simulink model "rtwdemo_roll_Step02a"  (R2022b)
settings: Solver=FixedStepDiscrete  StartTime=0.0  StopTime=30  FixedStep=0.025  RelTol=1e-3
model workspace (MATLAB code in the model file + MAT data in the model file):
  | cmdLim = Simulink.Parameter;
  | cmdLim.Value = 15;
  | cmdLim.Description = 'Limit for controlling the maximum surface command angle.';
  | cmdLim.Min = 0;
  | cmdLim.Max = 90;
  | cmdLim.DocUnits = 'deg';
  | 
  | dispGain = Simulink.Parameter;
  | dispGain.Value = 0.75;
  | dispGain.Description = 'Gain applied to the displacement error.';
  | dispGain.Min = 0;
  | dispGain.Max = [];
  | dispGain.DocUnits = 'deg/sec/deg';
  | 
  | dispLim = Simulink.Parameter;
  | dispLim.Value = 30;
  | dispLim.Description = 'Limit for controlling the maximum commanded angle.';
  | dispLim.Min = 0;
  | dispLim.Max = 180;
  | dispLim.DocUnits = 'deg';
  | 
  | intGain = Simulink.Parameter;
  | intGain.Value = 0.5;
  | intGain.Description = 'Gain applied to the integral error.';
  | intGain.Min = 0;
  | intGain.Max = [];
  | intGain.DocUnits = 'deg/sec/deg/sec';
  | 
  | intLim = Simulink.Parameter;
  | intLim.Value = 5;
  | intLim.Description = 'Limit for controlling the maximum commanded angle.';
  | intLim.Min = 0;
  | intLim.Max = 90;
  | intLim.DocUnits = 'deg';
  | 
  | rateGain = Simulink.Parameter;
  | rateGain.Value = 2;
  | rateGain.Description = 'Gain applied to the rate error.';
  | rateGain.Min = 0;
  | rateGain.Max = [];
  | rateGain.DocUnits = 'deg/deg/sec';
  | 
  | rateLim = Simulink.Parameter;
  | rateLim.Value = 6;
  | rateLim.Description = 'Limit for controlling the maximum commanded angle.';
  | rateLim.Min = 0;
  | rateLim.Max = 180;
  | rateLim.DocUnits = 'deg/sec';
  | 
  | hdgGain = Simulink.Parameter;
  | hdgGain.Value = 0.015;
undefined symbols (not defined in the file): DiscIntNeverNeededParam
libraries: simulink_need_slupdate x1
Description:
  | This model represents a basic roll axis autopilot with two operating
  | modes; roll attitude hold and heading hold. The mode logic for these
  | modes is external to this model.  The model architecture represents the
  | heading hold mode and basic roll attitude function as referenced models.
  | 
  | The roll attitude control function is a PID controller that uses roll
  | attitude and roll rate feedback to produce an aileron command.  The
  | input to the controller will be either a basic roll angle reference or a
  | roll command to track the desired heading.
settings Model: RequirementInfo={} %GIDa_fe9045fd_0412_4b6e_8206_617cc20e6fde  FPTRunName=Active  ModifiedByFormat=The MathWorks, Inc.  Creator=The MathWorks, Inc.  LastModifiedBy=The MathWorks, Inc.
settings SolverCC: AlgebraicLoopSolver=TrustRegion
settings DataIOCC: ExternalInput=xin  SaveFormat=StructureWithTime  SaveOutput=off  SignalLogging=off  DSMLogging=off  SaveTime=off  ReturnWorkspaceOutputs=off
settings OptimizationCC: UseDivisionForNetSlopeComputation=on  UseFloatMulNetSlope=on  EnhancedBackFolding=on  BooleansAsBitfields=on  PassReuseOutputArgsAs=Individual arguments  ExpressionDepthLimit=2147483647  NoFixptDivByZeroProtection=on  EfficientFloat2IntCast=on  MaxStackSize=inf  OptimizeBlockOrder=speed  DifferentSizesBufferReuse=on  EfficientTunableParamExpr=on
settings DebuggingCC: SignalRangeChecking=error  ReadBeforeWriteMsg=EnableAllAsError  WriteAfterWriteMsg=EnableAllAsError  WriteAfterReadMsg=EnableAllAsError  AlgebraicLoopMsg=error  ArtificialAlgebraicLoopMsg=error  SaveWithDisabledLinksMsg=error  SaveWithParameterizedLinksMsg=error  CheckExecutionContextPreStartOutputMsg=on  BlockPriorityViolationMsg=error  MaxConsecutiveZCsMsg=warning  SolverPrmCheckMsg=error  InheritedTsInSrcMsg=error  SingleTaskRateTransMsg=error  TasksWithSamePriorityMsg=error  SigSpecEnsureSampleTimeMsg=error  IntegerOverflowMsg=error  ParameterUnderflowMsg=error  ParameterPrecisionLossMsg=none  ParameterTunabilityLossMsg=error  UnderSpecifiedDataTypeMsg=error  UnnecessaryDatatypeConvMsg=warning  VectorMatrixConversionMsg=error  SignalLabelMismatchMsg=error  UnconnectedInputMsg=error  UnconnectedOutputMsg=error  UnconnectedLineMsg=error  SFcnCompatibilityMsg=error  UniqueDataStoreMsg=error  BusObjectLabelMismatch=error  RootOutportRequireBusObject=error  AssertControl=DisableAll  AllowSymbolicDim=off  ModelReferenceIOMsg=error  ModelReferenceIOMismatchMessage=error  UnknownTsInhSupMsg=error  ModelReferenceDataLoggingMessage=error  ModelReferenceSymbolNameMessage=none  ModelReferenceExtraNoncontSigs=none  StateNameClashWarn=warning  StrictBusMsg=ErrorOnBusTreatedAsVector  NonBusSignalsTreatedAsBus=error  SFInvalidInputDataAccessInChartInitDiag=error  SFTransitionOutsideNaturalParentDiag=error  SFUnreachableExecutionPathDiag=error  SFUndirectedBroadcastEventsDiag=error  SFExecutionAtInitializationDiag=none  SFMachineParentedDataDiag=warning  IntegerSaturationMsg=error  ArithmeticOperatorsInVariantConditions=warning
settings HardwareCC: ProdLongLongMode=on  TargetHWDeviceType=32-bit Generic
settings ModelReferenceCC: EnableRefExpFcnMdlSchedulingChecks=on  ModelReferenceNumInstancesAllowed=Single  PropagateSignalLabelsOutOfModel=off
settings SFSimCC: SimUseLocalCustomCode=off  MATLABDynamicMemAlloc=off
settings RTWCC: Description=Embedded Coder  SystemTargetFile=ert.tlc  GenCodeOnly=on  TemplateMakefile=ert_default_tmf  GenerateReport=on  RTWVerbose=off  RTWUseLocalCustomCode=off  CustomSource=roll_input_data.c  BuildConfiguration=Faster Runs  IncludeHyperlinkInReport=on  LaunchReport=on  GenerateTraceInfo=on  GenerateTraceReport=on  GenerateTraceReportSl=on  GenerateTraceReportSf=on  GenerateTraceReportEml=on  GenerateCodeMetricsReport=on  DLArmComputeVersion=19.05
settings CodeAppCC: ForceParamTrailComments=on  IgnoreCustomStorageClasses=off  OperatorAnnotations=on  SimulinkDataObjDesc=on  SFDataObjDesc=on  CustomSymbolStrGlobalVar=$N$M  CustomSymbolStrType=$N$M  CustomSymbolStrFcn=$N$M$F  CustomSymbolStrMacro=$N$M  InsertBlockDesc=on  ReqsInCode=on
settings ERTTargetCC: GenerateSampleERTMain=on  ERTCustomFileTemplate=example_file_process.tlc
settings ConfigComp: CovScope=ReferencedModels  CovSaveName=covdata_rollAP  CovMetricSettings=dcmtrwe  CovHTMLOptions=-sRT=1 -aTS=1 -bRG=1 -bTC=1 -hTR=1 -nFC=0 -scm=1 -bcm=1 -xEv=0  CovSaveCumulativeToWorkspaceVar=on  CovSaveSingleToWorkspaceVar=on  CovCumulativeVarName=covCumulativeData_rollAP  CovReportOnPause=off  CovExternalEMLEnable=off  CovSFcnEnable=off  DVModelCoverageObjectives=MCDC  DVMaxTestCaseSteps=500  DVTestSuiteOptimization=CombinedObjectives (Nonlinear Extended)  DVDetectActiveLogic=on  DVSaveHarnessModel=on  DVModelReferenceHarness=on  DVSaveReport=on  DVRebuildModelRepresentation=Always

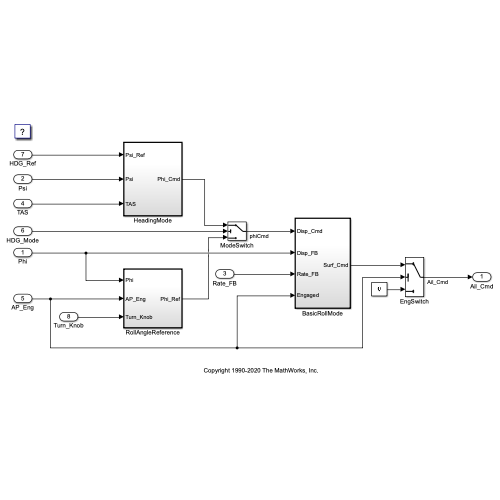
[thumbnail: Simulink's stored preview of the top-level diagram]
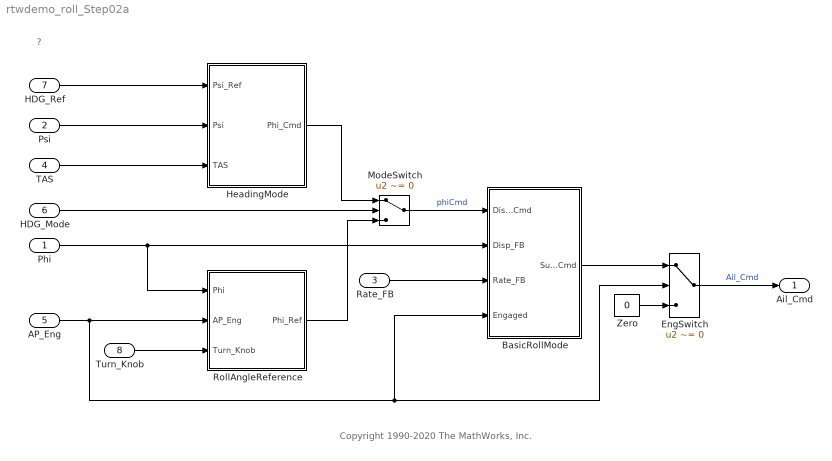
== system rtwdemo_roll_Step02a ==
  note: Copyright 1990-2020 The MathWorks, Inc.
  note: ?
  Phi : Inport  RequirementInfo={} %GIDa_040c2d73_6311_42f9_964f_56f1fff3d8d8  OutMin=-180  OutMax=180  OutDataTypeStr=single  PortDimensions=1  SampleTime=1/40  Interpolate=off
  Psi : Inport  RequirementInfo={} %GIDa_aa699f91_96f0_401b_acdb_f9b4b0743533  Port=2  OutMin=-180  OutMax=180  OutDataTypeStr=single  PortDimensions=1  SampleTime=1/40  Interpolate=off
  Rate_FB : Inport  RequirementInfo={} %GIDa_91b6e343_cedd_4c09_9e82_9cc09e4312a7  Port=3  OutMin=-60  OutMax=60  OutDataTypeStr=single  PortDimensions=1  SampleTime=1/40  Interpolate=off
  TAS : Inport  RequirementInfo={} %GIDa_9daa2c3d_09c1_4ac6_a206_1425f5f778cd  Port=4  OutMin=0  OutMax=1000  OutDataTypeStr=single  PortDimensions=1  SampleTime=1/40  Interpolate=off
  AP_Eng : Inport  RequirementInfo={} %GIDa_dbf8c750_871c_42fc_8ea1_57838e97fa97  Port=5  OutMin=0  OutMax=1  OutDataTypeStr=boolean  PortDimensions=1  SampleTime=1/40  Interpolate=off
  HDG_Mode : Inport  RequirementInfo={} %GIDa_3d1fd2be_b046_42ef_8f3c_1955bceadbb7  Port=6  OutMin=0  OutMax=1  OutDataTypeStr=boolean  PortDimensions=1  SampleTime=1/40  Interpolate=off
  HDG_Ref : Inport  RequirementInfo={} %GIDa_96162cda_cb1a_490e_8dac_f861526aad50  Port=7  OutMin=-180  OutMax=180  OutDataTypeStr=single  PortDimensions=1  SampleTime=1/40  Interpolate=off
  Turn_Knob : Inport  RequirementInfo={} %GIDa_fa976ccd_1ea9_4823_b673_fef2768ad601  Port=8  OutMin=-45  OutMax=45  OutDataTypeStr=single  PortDimensions=1  SampleTime=1/40  Interpolate=off
  BasicRollMode : Subsystem  TreatAsAtomicUnit=on
      settings: RTWSystemCode=Inline
  EngSwitch : Switch  RequirementInfo={} %GIDa_1f89e2a1_f10b_411b_80f1_4c7070559f04  Criteria=u2 ~= 0  OutDataTypeStr=single  SaturateOnIntegerOverflow=off  InputSameDT=off
  HeadingMode : Subsystem  TreatAsAtomicUnit=on
      settings: RTWSystemCode=Inline
  ModeSwitch : Switch  RequirementInfo={} %GIDa_89518de0_411a_4ee8_869d_c7ed5e5087e3  Criteria=u2 ~= 0  OutDataTypeStr=single  SaturateOnIntegerOverflow=off  InputSameDT=off
  RollAngleReference : Subsystem  RequirementInfo={} %GIDa_bf621fce_78e1_4f75_9fdb_aa952a465c6d  TreatAsAtomicUnit=on
      settings: RTWSystemCode=Inline
  Zero : Constant  RequirementInfo={} %GIDa_8c99e557_6257_4659_beae_770a67a6ac3a  Value=0  OutDataTypeStr=single
  Ail_Cmd : Outport  RequirementInfo={} %GIDa_02b61f6d_71d4_4b0d_89ac_bfbca808eb5f  OutMin=-15  OutMax=15  OutDataTypeStr=single  PortDimensions=1  SampleTime=1/40  VectorParamsAs1DForOutWhenUnconnected=off
  wires:
  HDG_Ref/1 -> HeadingMode/1(Psi_Ref)
  Phi/1 -> RollAngleReference/1(Phi), BasicRollMode/2(Disp_FB)
  Rate_FB/1 -> BasicRollMode/3(Rate_FB)
  Psi/1 -> HeadingMode/2(Psi)
  TAS/1 -> HeadingMode/3(TAS)
  ModeSwitch/1 -> BasicRollMode/1(Disp_Cmd)  "phiCmd"
  HDG_Mode/1 -> ModeSwitch/2
  HeadingMode/1(Phi_Cmd) -> ModeSwitch/1
  AP_Eng/1 -> BasicRollMode/4(Engaged), EngSwitch/2, RollAngleReference/2(AP_Eng)
  BasicRollMode/1(Surf_Cmd) -> EngSwitch/1
  EngSwitch/1 -> Ail_Cmd/1  "Ail_Cmd"
  Zero/1 -> EngSwitch/3
  RollAngleReference/1(Phi_Ref) -> ModeSwitch/3
  Turn_Knob/1 -> RollAngleReference/3(Turn_Knob)

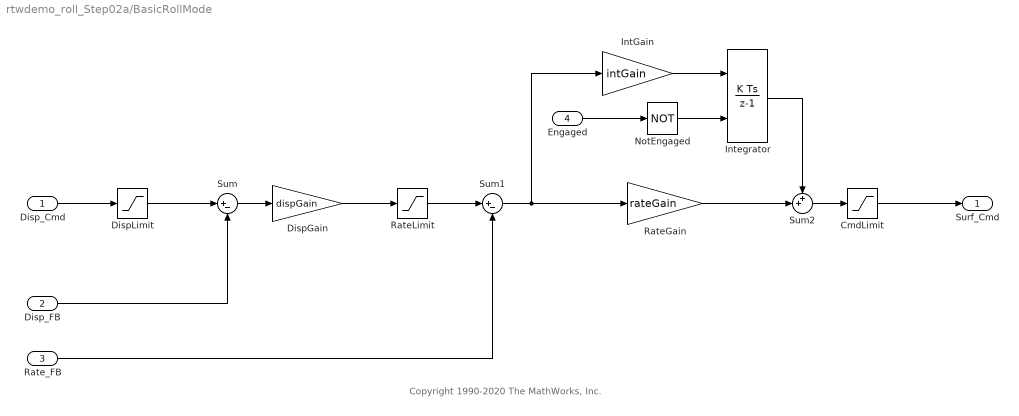
== system rtwdemo_roll_Step02a/BasicRollMode ==
  note: Copyright 1990-2020 The MathWorks, Inc.
  Disp_Cmd : Inport  RequirementInfo={} %GIDa_ff8f2950_36d2_4703_9842_3782e1cf4043  OutMin=-180  OutMax=180  OutDataTypeStr=single  PortDimensions=1  SampleTime=1/40
  Disp_FB : Inport  RequirementInfo={} %GIDa_88ab7783_4881_4494_98c7_fae9a40f845a  Port=2  OutMin=-180  OutMax=180  OutDataTypeStr=single  PortDimensions=1  SampleTime=1/40
  Rate_FB : Inport  RequirementInfo={} %GIDa_4b3300d7_83b5_4816_b86c_8919c709dd87  Port=3  OutMin=-60  OutMax=60  OutDataTypeStr=single  PortDimensions=1  SampleTime=1/40
  Engaged : Inport  RequirementInfo={} %GIDa_68912e61_3a66_45a7_b507_2a909d737c47  Port=4  OutMin=0  OutMax=1  OutDataTypeStr=boolean  PortDimensions=1  SampleTime=1/40
  CmdLimit : Saturate  RequirementInfo={} %GIDa_03acfcd2_0166_4b8d_8424_6cefd1433742  UpperLimit=cmdLim  LowerLimit=-cmdLim
      settings: AttributesFormatString=%<LowerLimit> to %<UpperLimit>\n(deg)
  DispGain : Gain  RequirementInfo={} %GIDa_dff0c99b_8bb2_4fb9_8fd5_e82c46b12065  Gain=dispGain  OutDataTypeStr=Inherit: Same as input  ParamDataTypeStr=Inherit: Same as input
  DispLimit : Saturate  RequirementInfo={} %GIDa_b12ad7d0_7f46_4ac9_8f07_3dc9a608e0b9  UpperLimit=dispLim  LowerLimit=-dispLim  OutMin=-dispLim  OutMax=dispLim
      settings: AttributesFormatString=%<LowerLimit> to %<UpperLimit>\n(deg)
  IntGain : Gain  RequirementInfo={} %GIDa_b5140734_8c8b_40a9_9825_d7d1205e8869  Gain=intGain  OutDataTypeStr=Inherit: Same as input  ParamDataTypeStr=Inherit: Same as input
  Integrator : DiscreteIntegrator  RequirementInfo={} %GIDa_4ed31261_78e4_4834_bce8_809b2d91a32f  ExternalReset=level  SampleTime=1/40  OutMin=-intLim  OutMax=intLim  OutDataTypeStr=single  LimitOutput=on  UpperSaturationLimit=intLim  LowerSaturationLimit=-intLim  IgnoreLimit=on  ICPrevOutput=DiscIntNeverNeededParam  ICPrevScaledInput=DiscIntNeverNeededParam
      settings: AttributesFormatString=%<LowerSaturationLimit> to %<UpperSaturationLimit> (deg)
  NotEngaged : Logic  RequirementInfo={} %GIDa_708249e7_acd0_4b17_bb48_cb1f255fa1ae  Operator=NOT  IconShape=distinctive  AllPortsSameDT=off  OutDataTypeStr=boolean
  RateGain : Gain  RequirementInfo={} %GIDa_1d522638_1084_40aa_a9e2_d20f3b201758  Gain=rateGain  OutDataTypeStr=Inherit: Same as input  ParamDataTypeStr=Inherit: Same as input
  RateLimit : Saturate  RequirementInfo={} %GIDa_3a07b6bd_f8e9_4edb_b789_30fb5da492d2  UpperLimit=rateLim  LowerLimit=-rateLim  OutMin=-rateLim  OutMax=rateLim
      settings: AttributesFormatString=%<LowerLimit> to %<UpperLimit>\n(deg/sec)
  Sum : Sum  RequirementInfo={} %GIDa_ed2635df_4414_4276_958f_e2737d50d7e7  Inputs=|+-  AccumDataTypeStr=single  OutDataTypeStr=single
  Sum1 : Sum  RequirementInfo={} %GIDa_c2525d12_4b8c_459a_a1b7_e9245b378d44  Inputs=|+-  AccumDataTypeStr=single  OutDataTypeStr=single
  Sum2 : Sum  RequirementInfo={} %GIDa_6cc23380_db4c_4d56_bea9_1d957a833aee  Inputs=++|  AccumDataTypeStr=single  OutDataTypeStr=single
  Surf_Cmd : Outport  RequirementInfo={} %GIDa_f913a5d7_0f1c_420b_9466_7f1cf663aa04  OutMin=-cmdLim  OutMax=cmdLim  OutDataTypeStr=single  PortDimensions=1  SampleTime=1/40  VectorParamsAs1DForOutWhenUnconnected=off
  wires:
  Disp_Cmd/1 -> DispLimit/1
  Disp_FB/1 -> Sum/2
  Rate_FB/1 -> Sum1/2
  Sum1/1 -> RateGain/1, IntGain/1
  DispGain/1 -> RateLimit/1
  Sum/1 -> DispGain/1
  DispLimit/1 -> Sum/1
  RateLimit/1 -> Sum1/1
  CmdLimit/1 -> Surf_Cmd/1
  RateGain/1 -> Sum2/2
  Sum2/1 -> CmdLimit/1
  Engaged/1 -> NotEngaged/1
  NotEngaged/1 -> Integrator/2
  Integrator/1 -> Sum2/1
  IntGain/1 -> Integrator/1

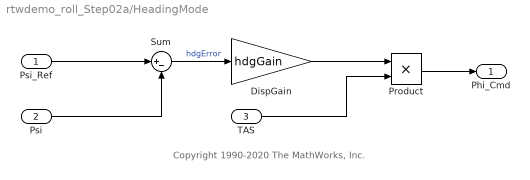
== system rtwdemo_roll_Step02a/HeadingMode ==
  note: Copyright 1990-2020 The MathWorks, Inc.
  Psi_Ref : Inport  RequirementInfo={} %GIDa_63217851_dfde_4515_9b44_03620ba74ebd  OutMin=-180  OutMax=180  OutDataTypeStr=single  PortDimensions=1  SampleTime=1/40  Interpolate=off
  Psi : Inport  RequirementInfo={} %GIDa_fd436e7a_0b55_4fc9_b9d1_7e931e78faf3  Port=2  OutMin=-180  OutMax=180  OutDataTypeStr=single  PortDimensions=1  SampleTime=1/40  Interpolate=off
  TAS : Inport  RequirementInfo={} %GIDa_5afcdc4c_2f58_40a9_83dd_f8ee574f1321  Port=3  OutMin=0  OutMax=1000  OutDataTypeStr=single  PortDimensions=1  SampleTime=1/40  Interpolate=off
  DispGain : Gain  RequirementInfo={} %GIDa_efcf24d9_d92c_4e12_9177_4c044d8f8aec  Gain=hdgGain  OutDataTypeStr=Inherit: Same as input  ParamDataTypeStr=Inherit: Same as input
  Product : Product  RequirementInfo={} %GIDa_7dbe21d3_99ef_4184_ab1e_23ac1efc2950  RndMeth=Zero  OutDataTypeStr=Inherit: Same as first input
  Sum : Sum  RequirementInfo={} %GIDa_3ad2d5f4_d194_4ab5_91b1_326f1f050e43  Inputs=|+-  OutDataTypeStr=Inherit: Same as first input
  Phi_Cmd : Outport  RequirementInfo={} %GIDa_6cfb4d70_f1fd_4187_9f6e_37a982bfddd8  OutDataTypeStr=single  PortDimensions=1  SampleTime=1/40  VectorParamsAs1DForOutWhenUnconnected=off
  wires:
  Product/1 -> Phi_Cmd/1
  DispGain/1 -> Product/1
  Sum/1 -> DispGain/1  "hdgError"
  Psi/1 -> Sum/2
  Psi_Ref/1 -> Sum/1
  TAS/1 -> Product/2

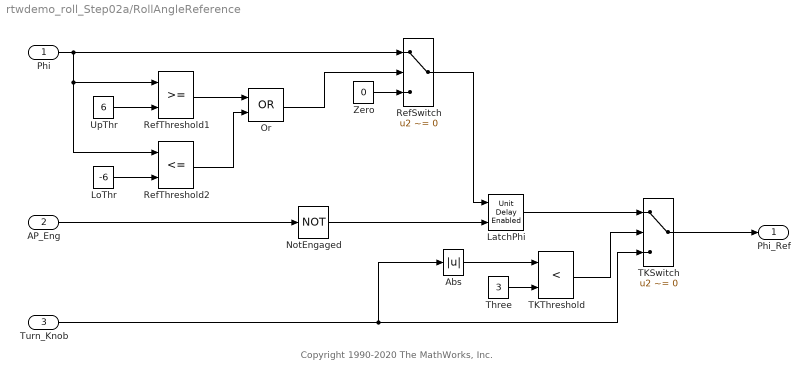
== system rtwdemo_roll_Step02a/RollAngleReference ==
  note: Copyright 1990-2020 The MathWorks, Inc.
  Phi : Inport  RequirementInfo={} %GIDa_9b709a66_f791_47f7_86bd_e175ebb7b1b4  OutDataTypeStr=single
  AP_Eng : Inport  RequirementInfo={} %GIDa_9de52ebb_3f37_4f5e_876e_6853370267c1  Port=2  OutDataTypeStr=boolean
  Turn_Knob : Inport  RequirementInfo={} %GIDa_fcc46fb4_e425_442f_ac5c_e3f314b4cbdd  Port=3  OutDataTypeStr=single
  Abs : Abs  RequirementInfo={} %GIDa_daf2388c_0592_4fd8_9932_fc6ad2b28c75  SaturateOnIntegerOverflow=off
  LatchPhi : simulink_need_slupdate/Unit Delay Enabled  RequirementInfo={} %GIDa_8c2a6474_62f7_4673_9b80_815aaee792d7  vinit=0.0  tsamp=1/40
  LoThr : Constant  RequirementInfo={} %GIDa_3d290e71_7846_48ec_bba2_120ec195a4d2  Value=-6  OutDataTypeStr=single
  NotEngaged : Logic  RequirementInfo={} %GIDa_e52c6893_d81b_4f15_89c3_12b6a83c27b2  Operator=NOT  IconShape=distinctive  AllPortsSameDT=off  OutDataTypeStr=boolean
  Or : Logic  RequirementInfo={} %GIDa_5a2f4265_d6d2_48b0_88b1_9f813e67f638  Operator=OR  OutDataTypeStr=boolean
  RefSwitch : Switch  RequirementInfo={} %GIDa_a4746381_6ebe_4e3d_83b9_b49d14a3af5e  Criteria=u2 ~= 0  OutDataTypeStr=single  SaturateOnIntegerOverflow=off  InputSameDT=off
  RefThreshold1 : RelationalOperator  RequirementInfo={} %GIDa_be19764a_4253_499a_816c_5a218f85ba52  OutDataTypeStr=boolean
  RefThreshold2 : RelationalOperator  RequirementInfo={} %GIDa_66db49a9_aa40_43ab_9d6f_efe68ac443ed  Operator=<=  OutDataTypeStr=boolean
  TKSwitch : Switch  RequirementInfo={} %GIDa_804165d0_89eb_4919_a8d1_f2310004f7d9  Criteria=u2 ~= 0  OutDataTypeStr=single  SaturateOnIntegerOverflow=off  InputSameDT=off
  TKThreshold : RelationalOperator  RequirementInfo={} %GIDa_9859b478_272f_4974_a36c_6c4f8c030643  Operator=<  OutDataTypeStr=boolean
  Three : Constant  RequirementInfo={} %GIDa_6228e2c4_8022_4eaf_90d6_7c47f19fb0a2  Value=3  OutDataTypeStr=single
  UpThr : Constant  RequirementInfo={} %GIDa_0870d8d6_d29f_4cb4_9c0c_9079ccdb7173  Value=6  OutDataTypeStr=single
  Zero : Constant  RequirementInfo={} %GIDa_e4775650_e5c7_4c74_aef4_71c144af3cbc  Value=0  OutDataTypeStr=single
  Phi_Ref : Outport  RequirementInfo={} %GIDa_130f2b33_9208_4d69_9109_0436e6034ad0  OutMin=-180  OutMax=180  OutDataTypeStr=single  VectorParamsAs1DForOutWhenUnconnected=off
  wires:
  NotEngaged/1 -> LatchPhi/2
  RefSwitch/1 -> LatchPhi/1
  LatchPhi/1 -> TKSwitch/1
  TKThreshold/1 -> TKSwitch/2
  Turn_Knob/1 -> TKSwitch/3, Abs/1
  Three/1 -> TKThreshold/2
  Abs/1 -> TKThreshold/1
  Phi/1 -> RefSwitch/1, RefThreshold1/1, RefThreshold2/1
  AP_Eng/1 -> NotEngaged/1
  TKSwitch/1 -> Phi_Ref/1
  UpThr/1 -> RefThreshold1/2
  Zero/1 -> RefSwitch/3
  Or/1 -> RefSwitch/2
  RefThreshold1/1 -> Or/1
  RefThreshold2/1 -> Or/2
  LoThr/1 -> RefThreshold2/2
